simulink model "power_ForwardConverter"  (R2018a)
settings: Solver=VariableStepAuto  StartTime=0.0  StopTime=0.013  MaxStep=1e-4  RelTol=1e-4  EnableMultiTasking=on
libraries: powerlib x15
Description:
  | Copyright 2008-2018 The MathWorks, Inc.
settings Model: Creator=MathWorks  LastModifiedBy=rmkna
settings SolverCC: SolverResetMethod=Robust
settings DataIOCC: ReturnWorkspaceOutputs=on
settings OptimizationCC: LifeSpan=inf
settings DebuggingCC: ReadBeforeWriteMsg=DisableAll  WriteAfterWriteMsg=DisableAll  WriteAfterReadMsg=DisableAll  MultiTaskDSMMsg=none  SFUnexpectedBacktrackingDiag=warning  SFNoUnconditionalDefaultTransitionDiag=warning  SFExecutionAtInitializationDiag=none
settings ModelReferenceCC: UpdateModelReferenceTargets=IfOutOfDate
settings SFSimCC: SFSimEcho=off
settings CodeAppCC: StateflowObjectComments=on
settings GRTTargetCC: TargetLangStandard=C89/C90 (ANSI)  GeneratePreprocessorConditionals=Disable all
settings ConfigComp: CovMetricSettings=dw  CovHtmlReporting=on  CovSaveCumulativeToWorkspaceVar=on  CovSaveSingleToWorkspaceVar=on  CovExternalEMLEnable=off
settings SimscapeCC: SimscapeNormalizeSystem=off  SimscapeNominalValues={1, 'bar'; 1, 'cm^3/s'; 1, 'bar*kg/s'; 1, 'kJ/kg'; 1, 'kW'; }

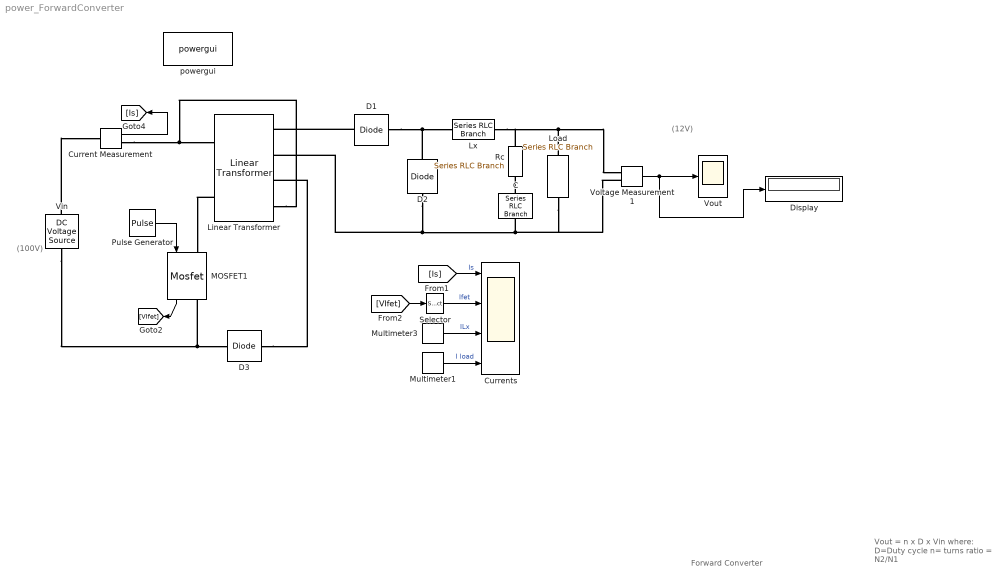
== system power_ForwardConverter ==
  note: (12V)
  note: Vout = n x D x Vin
      | where: D=Duty cycle
      | n= turns ratio = N2/N1
  note: (100V)
  note: Forward Converter
  C : powerlib/Elements/Series RLC Branch  LConnTagsString=__new0  RConnTagsString=__new0  BranchType=C  Resistance=1e-4  Inductance=200e-6  SetiL0=off  InitialCurrent=0  Capacitance=100e-6  Setx0=off  InitialVoltage=0  Measurements=None
  Current Measurement : powerlib/Measurements/Current Measurement  PhasorSimulation=off  OutputType=Complex  PSBequivalent=0
  Currents : Scope  NumInputPorts=4
  D1 : powerlib/Power Electronics/Diode  Ron=1e-3  Lon=0  Vf=0.7  IC=0  UseSnubber=off  Rs=inf  Cs=0  Measurements=off
  D2 : powerlib/Power Electronics/Diode  Ron=1e-3  Lon=0  Vf=0.7  IC=0  UseSnubber=off  Rs=inf  Cs=0  Measurements=off
  D3 : powerlib/Power Electronics/Diode  Ron=1e-3  Lon=0  Vf=0.8  IC=0  UseSnubber=off  Rs=inf  Cs=0  Measurements=off
  Display : Display
  Linear Transformer : powerlib/Elements/Linear Transformer  UNITS=SI  NominalPower=[ 50 100e3 ]  winding1=[100 0 0]  winding2=[25 0 0]  ThreeWindings=on  winding3=[100 0 0]  RmLm=[inf 10e-3]  Measurements=Magnetization current  DataType=on
  Load : powerlib/Elements/Series RLC Branch  LConnTagsString=__new0  RConnTagsString=__new0  BranchType=R  Resistance=2.8  Inductance=200e-6  SetiL0=off  InitialCurrent=0  Capacitance=400e-6  Setx0=off  InitialVoltage=0  Measurements=Branch current
  Lx : powerlib/Elements/Series RLC Branch  LConnTagsString=__new0  RConnTagsString=__new0  BranchType=L  Resistance=10  Inductance=50e-6  SetiL0=off  InitialCurrent=0  Capacitance=400e-6  Setx0=off  InitialVoltage=0  Measurements=Branch current
  MOSFET1 : powerlib/Power Electronics/Mosfet  Ron=1e-3  Lon=0  Rd=1e-3  Vfd=0  IC=0  Rs=1e6  Cs=inf  Measurements=on
  Multimeter1 : powerlib/Measurements/Multimeter  PhasorSimulation=off  OutputType=Complex  sel=1  L=6  Gain=1  yselected={'Ib: Load'};  PSBOutputType=1  PSBequivalent=0  AxesSetting=[0,0.1,-100,100]  Display=0  SavedBlockNames=-11
  Multimeter3 : powerlib/Measurements/Multimeter  PhasorSimulation=off  OutputType=Complex  sel=2  L=6  Gain=1  yselected={'Ib: Lx'};  PSBOutputType=1  PSBequivalent=0  AxesSetting=[0,0.1,-100,100]  Display=0  SavedBlockNames=-11
  Pulse Generator : DiscretePulseGenerator  PulseType=Time based  Period=1/100e3  PulseWidth=50
  Rc : powerlib/Elements/Series RLC Branch  LConnTagsString=__new0  RConnTagsString=__new0  BranchType=R  Resistance=50e-3  Inductance=200e-6  SetiL0=off  InitialCurrent=0  Capacitance=400e-6  Setx0=off  InitialVoltage=0  Measurements=Branch current
  Selector : Selector  InputPortWidth=2  IndexOptions=Index vector (dialog)  Indices=1  OutputSizes=1
  Vin : powerlib/Electrical Sources/DC Voltage Source  Amplitude=100  Measurements=None
  Voltage Measurement1 : powerlib/Measurements/Voltage Measurement  PhasorSimulation=off  OutputType=Complex  PSBequivalent=0
  Vout : Scope
  powergui : powerlib/powergui  Priority=1  SimulationMode=Continuous  SampleTime=50e-6  frequency=60  Iterations=50  frequencyindice=0  Pbase=100e6  ErrMax=1e-4  UnitsV=kV  UnitsW=MW  buscounter=0  FunctionMessages=off  echomessages=off  EnableUseOfTLC=off  CurrentSourceSwitches=off  DisableSnubberDevices=off  DisableRonSwitches=off  DisableVfSwitches=off  DisplayEquations=off  SolverType=Tustin/Backward Euler (TBE)  Interpol=off  ExternalGateDelay=off  methode=off  Ts=100  x0status=blocks  SPID=on  SwTol=0  HookPort=off  RestoreLinks=warning  ResistiveCurrentMeasurement=off  Frange=[0:2:500]  Ylog=off  Xlog=on  ShowGrid=off  save=off  variable=ZData  structure=0  ZoomFFT=off  StartTime=0.0  cycles=1  DisplayStyle=1  fundamental=60  FreqAxis=off  MaxFrequency=1000  frequencyindicesteady=1  RmsSteady=1  display=off
  wires:
  MOSFET1/1 -> [VIfet]
  [VIfet] -> Selector/1
  Current Measurement/1 -> [Is]
  [Is] -> Currents/1  "Is"
  Multimeter3/1 -> Currents/3  "ILx"
  Selector/1 -> Currents/2  "Ifet"
  Voltage Measurement1/1 -> Display/1, Vout/1
  Pulse Generator/1 -> MOSFET1/1
  Multimeter1/1 -> Currents/4  "I load"
  connections:
  Rc/LConn1 -- Lx/RConn1 -- Load/LConn1 -- Voltage Measurement1/LConn1
  D2/LConn1 -- C/RConn1 -- Load/RConn1 -- Voltage Measurement1/LConn2 -- Linear Transformer/RConn2
  Linear Transformer/LConn2 -- MOSFET1/LConn1
  Vin/LConn1 -- D3/LConn1 -- MOSFET1/RConn1
  Linear Transformer/RConn4 -- Current Measurement/RConn1 -- Linear Transformer/LConn1
  D1/LConn1 -- Linear Transformer/RConn1
  D2/RConn1 -- D1/RConn1 -- Lx/LConn1
  D3/RConn1 -- Linear Transformer/RConn3
  Vin/RConn1 -- Current Measurement/LConn1
  C/LConn1 -- Rc/RConn1
